simulink model "PlantPan"  (Simulink 6.1)
settings: Solver=ode45  StartTime=0.0  StopTime=1/testFreq*5  RelTol=1e-3
values from neighbouring files (symbols this model uses):
  delayInquiryPan = .015    (= 0.015)    [simPan.m]
  periodPanControl = periodFrame * framesPerPan    (= 0.066)    [simPan.m]
  pPan = 1/(1+s/15)^2    [simPan.m]
  rateLimitPan = 290    [simPan.m]
settings Model: LastModifiedBy=Big E
settings DebuggingCC: SolverPrmCheckMsg=warning

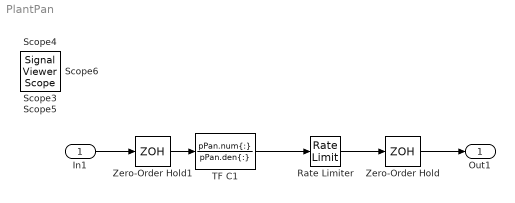
== system PlantPan ==
  In1 : Inport  Port=1  LatchInput=off
  Rate Limiter : RateLimiter  RisingSlewLimit=rateLimitPan  FallingSlewLimit=-rateLimitPan  SampleTimeMode=inherited
  TF C1 : TransferFcn  Numerator=pPan.num{:}  Denominator=pPan.den{:}
  Zero-Order Hold : ZeroOrderHold  SampleTime=delayInquiryPan
  Zero-Order Hold1 : ZeroOrderHold  SampleTime=periodPanControl
  Out1 : Outport
  Scope{3..6} (4 alike) : SignalViewerScope  IOType=viewer  RefreshTime=0.035000
  wires:
  In1/1 -> Zero-Order Hold1/1
  Zero-Order Hold1/1 -> TF C1/1
  Zero-Order Hold/1 -> Out1/1
  Rate Limiter/1 -> Zero-Order Hold/1
  TF C1/1 -> Rate Limiter/1
